simulink library "INT_Rail_SetPointCor"  (R2016b)
settings: Solver=VariableStepAuto  StartTime=0.0  StopTime=10.0  RelTol=1e-3
settings Model: Creator=mayongchao  LastModifiedBy=mayongchao

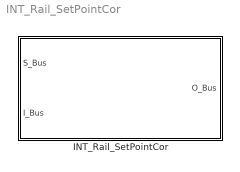
== system INT_Rail_SetPointCor ==
  INT_Rail_SetPointCor : Subsystem

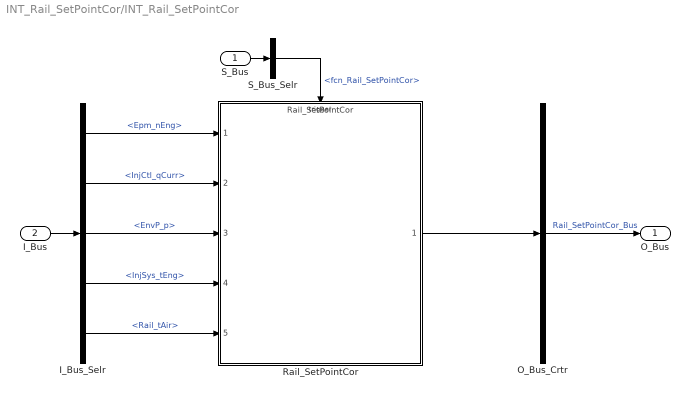
== system INT_Rail_SetPointCor/INT_Rail_SetPointCor ==
  S_Bus : Inport
  I_Bus : Inport  Port=2
  I_Bus_Selr : BusSelector  OutputSignals=Epm_nEng,InjCtl_qCurr,EnvP_p,InjSys_tEng,Rail_tAir
  O_Bus_Crtr : BusCreator  Inputs=1
  Rail_SetPointCor : ModelReference  ModelNameDialog=Rail_SetPointCor  SimulationMode=Normal  ModelReferenceVersion=1.15  TriggerPortName=function  TriggerPortTriggerType=function-call  TriggerPortStatesWhenEnabling=held
  S_Bus_Selr : BusSelector  OutputSignals=fcn_Rail_SetPointCor
  O_Bus : Outport
  wires:
  S_Bus_Selr/1 -> Rail_SetPointCor/Trigger  "<fcn_Rail_SetPointCor>"
  S_Bus/1 -> S_Bus_Selr/1
  I_Bus/1 -> I_Bus_Selr/1
  I_Bus_Selr/1 -> Rail_SetPointCor/1  "<Epm_nEng>"
  I_Bus_Selr/2 -> Rail_SetPointCor/2  "<InjCtl_qCurr>"
  I_Bus_Selr/3 -> Rail_SetPointCor/3  "<EnvP_p>"
  I_Bus_Selr/4 -> Rail_SetPointCor/4  "<InjSys_tEng>"
  I_Bus_Selr/5 -> Rail_SetPointCor/5  "<Rail_tAir>"
  O_Bus_Crtr/1 -> O_Bus/1  "Rail_SetPointCor_Bus"
  Rail_SetPointCor/1 -> O_Bus_Crtr/1
